simulink model "fec_ber_hw_V2"  (R2020b)
settings: Solver=FixedStepDiscrete  StartTime=0.0  StopTime=T  RelTol=1e-3
values from neighbouring files (symbols this model uses):
  aximm_awgn_reset = 0    [setup.m]
  aximm_bit_count_reset = 0    [setup.m]
  aximm_bits = n_blocks * k    (= 80)    [setup.m]
  aximm_ctrl_word_dec = 0    [setup.m]
  aximm_ctrl_word_enc = 0    [setup.m]
  aximm_enable = 1    [setup.m]
  aximm_length = k * n_blocks    (= 80)    [setup.m]
  aximm_length_dec = n    (= 160)    [setup.m]
  aximm_length_enc = k    (= 80)    [setup.m]
  aximm_llr_mag_reset = 0    [setup.m]
  aximm_llr_scale = (1/noise_var) * llr_scale    (= 1000)    [setup.m]
  aximm_load_dec = 1    [setup.m]
  aximm_load_enc = 1    [setup.m]
  aximm_noise_std = sqrt(noise_var)    [setup.m]
  aximm_reset = 0    [setup.m]
  d = sqrt(-2*log([0:1/4095:1]))    [setup.m]
  fs = 160e6    (= 160000000)    [setup.m]
  generator_polynomial = '''z^13 + z^12 + z^11 + z^8 + 1'''    [setup.m]
  llr_scale = 7.75/7.75    (= 1)    [setup.m]
libraries: simulink x931, hdlsllib x419, commseqgen3 x52, dspsigops x22, commblkcod2 x3, lib_rfsoc_fec x2
(part 4 of 47)

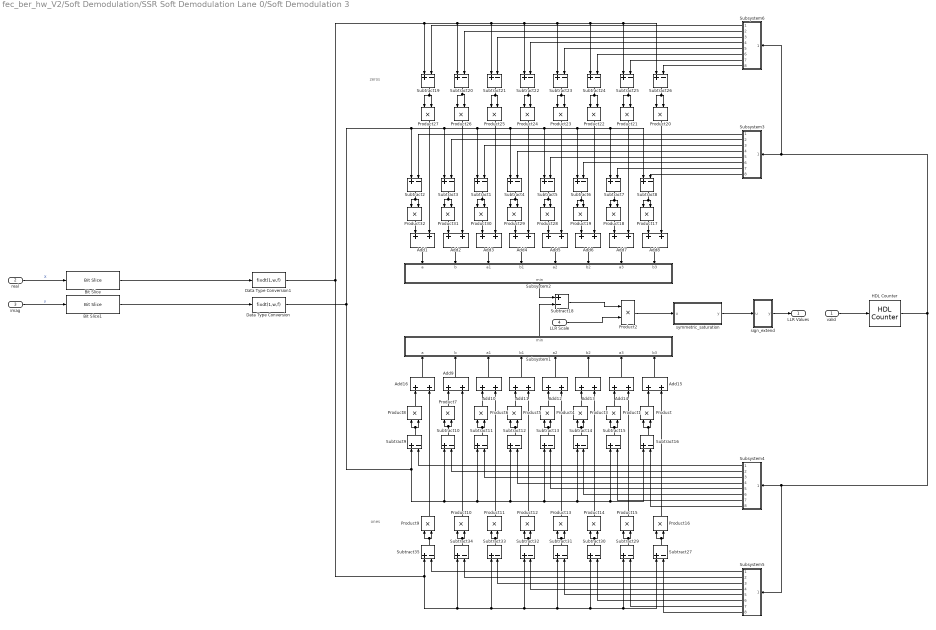
== system fec_ber_hw_V2/Soft Demodulation/SSR Soft Demodulation Lane 0/Soft Demodulation 3 ==
  note: ones
  note: zeros
  valid : Inport
  real : Inport  Port=2
  imag : Inport  Port=3
  LLR Scale : Inport  Port=4
  Add{1..16} (16 alike) : Sum  OutDataTypeStr=fixdt(1,(w+1)*2+1,f*2)  SaturateOnIntegerOverflow=on
  Bit Slice : hdlsllib/Logic and Bit Operations/Bit Slice  lidx=(n*w)-1  ridx=(n-1)*w
      settings: SourceProductBaseCode=SL
  Bit Slice1 : hdlsllib/Logic and Bit Operations/Bit Slice  lidx=(n*w)-1  ridx=(n-1)*w
      settings: SourceProductBaseCode=SL
  Data Type Conversion : DataTypeConversion  OutDataTypeStr=fixdt(1,w,f)  ConvertRealWorld=Stored Integer (SI)
  Data Type Conversion1 : DataTypeConversion  OutDataTypeStr=fixdt(1,w,f)  ConvertRealWorld=Stored Integer (SI)
  HDL Counter : hdlsllib/Sources/HDL Counter  CountType=Count limited  CountInit=0  CountStep=1  CountMax=3  CountFromType=Initial value  CountFrom=0  CountResetPort=off  CountLoadPort=off  CountEnbPort=on  CountDirPort=off  CountDataType=Unsigned  CountWordLen=2  CountFracLen=0  CountSampTime=1/(fs*2)
  Product{,1,3..16} (16 alike) : Product  SaturateOnIntegerOverflow=on
  Product{17..32} (16 alike) : Product
  Product2 : Product  RndMeth=Round  SaturateOnIntegerOverflow=on
  Subsystem1 : Subsystem
  Subsystem2 : Subsystem
  Subsystem3 : Subsystem
  Subsystem4 : Subsystem
  Subsystem5 : Subsystem
  Subsystem6 : Subsystem
  Subtract{1..16,19..27,29..35} (32 alike) : Sum  Inputs=+-  OutDataTypeStr=fixdt(1,w+1,f)  SaturateOnIntegerOverflow=on
  Subtract18 : Sum  Inputs=+-  OutDataTypeStr=fixdt(1,(w+1)*2+2,f*2)  SaturateOnIntegerOverflow=on
  sign_extend : Subsystem
  symmetric_saturation : MATLAB Function  TreatAsAtomicUnit=on
  LLR Values : Outport
  wires:
  Bit Slice/1 -> Data Type Conversion1/1
  Bit Slice1/1 -> Data Type Conversion/1
  Data Type Conversion1/1 -> Subtract27/1, Subtract29/1, Subtract30/1, Subtract31/1, Subtract32/1, Subtract33/1, Subtract34/1, Subtract35/1, Subtract20/1, Subtract26/1, Subtract25/1, Subtract24/1, Subtract23/1, Subtract22/1, Subtract21/1, Subtract19/1
  Data Type Conversion/1 -> Subtract15/1, Subtract16/1, Subtract14/1, Subtract13/1, Subtract12/1, Subtract11/1, Subtract10/1, Subtract9/1, Subtract7/1, Subtract8/1, Subtract6/1, Subtract5/1, Subtract4/1, Subtract1/1, Subtract3/1, Subtract2/1
  sign_extend/1(y) -> LLR Values/1
  Product2/1 -> symmetric_saturation/1(u)
  symmetric_saturation/1(y) -> sign_extend/1(u)
  HDL Counter/1 -> Subsystem3/1(enb), Subsystem6/1(enb), Subsystem4/1(enb), Subsystem5/1(enb)
  valid/1 -> HDL Counter/1
  Subsystem6/8(Out8) -> Subtract26/2
  Subsystem6/7(Out7) -> Subtract25/2
  Subsystem6/6(Out6) -> Subtract24/2
  Subsystem6/5(Out5) -> Subtract23/2
  Subsystem6/4(Out4) -> Subtract22/2
  Subsystem6/3(Out3) -> Subtract21/2
  Subsystem6/2(Out2) -> Subtract20/2
  Subsystem6/1(Out1) -> Subtract19/2
  Subtract6/1 -> Product19/2, Product19/1
  Subtract22/1 -> Product24/2, Product24/1
  Subtract20/1 -> Product26/1, Product26/2
  Subtract7/1 -> Product18/2, Product18/1
  Subtract8/1 -> Product17/1, Product17/2
  Subtract27/1 -> Product16/2, Product16/1
  Subtract29/1 -> Product15/2, Product15/1
  Subtract30/1 -> Product14/2, Product14/1
  Subtract31/1 -> Product13/2, Product13/1
  Subtract32/1 -> Product12/2, Product12/1
  Subtract33/1 -> Product11/2, Product11/1
  Subtract14/1 -> Product3/2, Product3/1
  Subsystem5/5(Out5) -> Subtract31/2
  Subtract16/1 -> Product/1, Product/2
  Add5/1 -> Subsystem2/5(a2)
  Subsystem3/8(Out8) -> Subtract8/2
  Add4/1 -> Subsystem2/4(b1)
  Product11/1 -> Add10/2
  Product29/1 -> Add4/1
  Subsystem4/8(Out8) -> Subtract16/2
  Subsystem4/2(Out2) -> Subtract10/2
  Subsystem5/8(Out8) -> Subtract27/2
  Subsystem5/7(Out7) -> Subtract29/2
  Subtract11/1 -> Product6/1, Product6/2
  Subtract34/1 -> Product10/1, Product10/2
  Product32/1 -> Add1/1
  Subsystem5/1(Out1) -> Subtract35/2
  Subtract12/1 -> Product5/1, Product5/2
  Subsystem3/7(Out7) -> Subtract7/2
  Product16/1 -> Add15/2
  Subsystem4/1(Out1) -> Subtract9/2
  Subsystem5/6(Out6) -> Subtract30/2
  Product24/1 -> Add4/2
  Subtract3/1 -> Product31/2, Product31/1
  Product13/1 -> Add12/2
  Subsystem5/3(Out3) -> Subtract33/2
  Subsystem5/2(Out2) -> Subtract34/2
  Subsystem4/3(Out3) -> Subtract11/2
  Product17/1 -> Add8/1
  Subsystem4/4(Out4) -> Subtract12/2
  Product9/1 -> Add16/2
  Add9/1 -> Subsystem1/2(b)
  Subsystem4/7(Out7) -> Subtract15/2
  Subtract26/1 -> Product20/2, Product20/1
  Subsystem3/3(Out3) -> Subtract1/2
  Product28/1 -> Add5/1
  Product12/1 -> Add11/2
  Product8/1 -> Add16/1
  Product7/1 -> Add9/1
  Subsystem4/5(Out5) -> Subtract13/2
  Subsystem3/4(Out4) -> Subtract4/2
  Product21/1 -> Add7/2
  Subtract25/1 -> Product21/2, Product21/1
  Add6/1 -> Subsystem2/6(b2)
  Add11/1 -> Subsystem1/4(b1)
  Add2/1 -> Subsystem2/2(b)
  Product15/1 -> Add14/2
  Product14/1 -> Add13/2
  Add8/1 -> Subsystem2/8(b3)
  Product27/1 -> Add1/2
  Subsystem3/1(Out1) -> Subtract2/2
  Subtract9/1 -> Product8/1, Product8/2
  Subtract15/1 -> Product1/1, Product1/2
  Subtract23/1 -> Product23/1, Product23/2
  Add14/1 -> Subsystem1/7(a3)
  imag/1 -> Bit Slice1/1  "y"
  Add16/1 -> Subsystem1/1(a)
  Subtract2/1 -> Product32/2, Product32/1
  Subtract5/1 -> Product28/2, Product28/1
  Subtract4/1 -> Product29/1, Product29/2
  Product18/1 -> Add7/1
  Add15/1 -> Subsystem1/8(b3)
  Product30/1 -> Add3/1
  Subsystem3/5(Out5) -> Subtract5/2
  Product31/1 -> Add2/1
  Subtract19/1 -> Product27/2, Product27/1
  Product26/1 -> Add2/2
  Add13/1 -> Subsystem1/6(b2)
  Subsystem3/2(Out2) -> Subtract3/2
  Product22/1 -> Add6/2
  Subsystem1/1(min) -> Subtract18/2
  Product5/1 -> Add11/1
  Subtract18/1 -> Product2/1
  Subsystem4/6(Out6) -> Subtract14/2
  Subtract1/1 -> Product30/2, Product30/1
  Subtract24/1 -> Product22/2, Product22/1
  Add10/1 -> Subsystem1/3(a1)
  LLR Scale/1 -> Product2/2
  Product4/1 -> Add12/1
  Subtract21/1 -> Product25/2, Product25/1
  Product23/1 -> Add5/2
  Add7/1 -> Subsystem2/7(a3)
  Product3/1 -> Add13/1
  Product19/1 -> Add6/1
  Product25/1 -> Add3/2
  real/1 -> Bit Slice/1  "X"
  Subtract35/1 -> Product9/1, Product9/2
  Subtract10/1 -> Product7/1, Product7/2
  Subsystem3/6(Out6) -> Subtract6/2
  Subsystem2/1(min) -> Subtract18/1
  Add3/1 -> Subsystem2/3(a1)
  Product20/1 -> Add8/2
  Add1/1 -> Subsystem2/1(a)
  Product/1 -> Add15/1
  Subtract13/1 -> Product4/2, Product4/1
  Product1/1 -> Add14/1
  Add12/1 -> Subsystem1/5(a2)
  Product10/1 -> Add9/2
  Product6/1 -> Add10/1
  Subsystem5/4(Out4) -> Subtract32/2

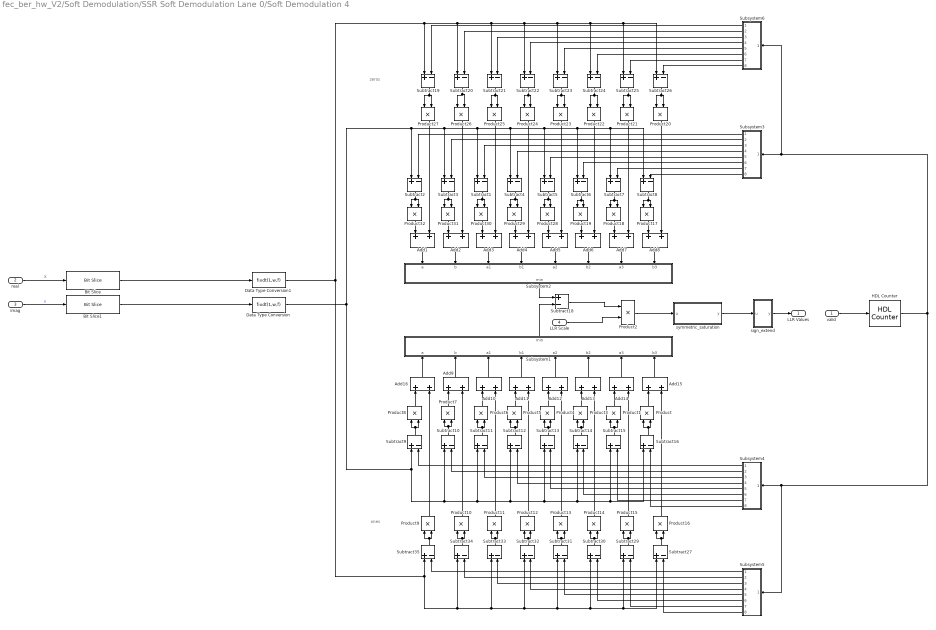
== system fec_ber_hw_V2/Soft Demodulation/SSR Soft Demodulation Lane 0/Soft Demodulation 4 ==
  note: ones
  note: zeros
  valid : Inport
  real : Inport  Port=2
  imag : Inport  Port=3
  LLR Scale : Inport  Port=4
  Add{1..16} (16 alike) : Sum  OutDataTypeStr=fixdt(1,(w+1)*2+1,f*2)  SaturateOnIntegerOverflow=on
  Bit Slice : hdlsllib/Logic and Bit Operations/Bit Slice  lidx=(n*w)-1  ridx=(n-1)*w
      settings: SourceProductBaseCode=SL
  Bit Slice1 : hdlsllib/Logic and Bit Operations/Bit Slice  lidx=(n*w)-1  ridx=(n-1)*w
      settings: SourceProductBaseCode=SL
  Data Type Conversion : DataTypeConversion  OutDataTypeStr=fixdt(1,w,f)  ConvertRealWorld=Stored Integer (SI)
  Data Type Conversion1 : DataTypeConversion  OutDataTypeStr=fixdt(1,w,f)  ConvertRealWorld=Stored Integer (SI)
  HDL Counter : hdlsllib/Sources/HDL Counter  CountType=Count limited  CountInit=0  CountStep=1  CountMax=3  CountFromType=Initial value  CountFrom=0  CountResetPort=off  CountLoadPort=off  CountEnbPort=on  CountDirPort=off  CountDataType=Unsigned  CountWordLen=2  CountFracLen=0  CountSampTime=1/(fs*2)
  Product{,1,3..16} (16 alike) : Product  SaturateOnIntegerOverflow=on
  Product{17..32} (16 alike) : Product
  Product2 : Product  RndMeth=Round  SaturateOnIntegerOverflow=on
  Subsystem1 : Subsystem
  Subsystem2 : Subsystem
  Subsystem3 : Subsystem
  Subsystem4 : Subsystem
  Subsystem5 : Subsystem
  Subsystem6 : Subsystem
  Subtract{1..16,19..27,29..35} (32 alike) : Sum  Inputs=+-  OutDataTypeStr=fixdt(1,w+1,f)  SaturateOnIntegerOverflow=on
  Subtract18 : Sum  Inputs=+-  OutDataTypeStr=fixdt(1,(w+1)*2+2,f*2)  SaturateOnIntegerOverflow=on
  sign_extend : Subsystem
  symmetric_saturation : MATLAB Function  TreatAsAtomicUnit=on
  LLR Values : Outport
  wires:
  Bit Slice/1 -> Data Type Conversion1/1
  Bit Slice1/1 -> Data Type Conversion/1
  Data Type Conversion1/1 -> Subtract27/1, Subtract29/1, Subtract30/1, Subtract31/1, Subtract32/1, Subtract33/1, Subtract34/1, Subtract35/1, Subtract20/1, Subtract26/1, Subtract25/1, Subtract24/1, Subtract23/1, Subtract22/1, Subtract21/1, Subtract19/1
  Data Type Conversion/1 -> Subtract15/1, Subtract16/1, Subtract14/1, Subtract13/1, Subtract12/1, Subtract11/1, Subtract10/1, Subtract9/1, Subtract7/1, Subtract8/1, Subtract6/1, Subtract5/1, Subtract4/1, Subtract1/1, Subtract3/1, Subtract2/1
  sign_extend/1(y) -> LLR Values/1
  Product2/1 -> symmetric_saturation/1(u)
  symmetric_saturation/1(y) -> sign_extend/1(u)
  HDL Counter/1 -> Subsystem3/1(enb), Subsystem6/1(enb), Subsystem4/1(enb), Subsystem5/1(enb)
  valid/1 -> HDL Counter/1
  Subsystem6/8(Out8) -> Subtract26/2
  Subsystem6/7(Out7) -> Subtract25/2
  Subsystem6/6(Out6) -> Subtract24/2
  Subsystem6/5(Out5) -> Subtract23/2
  Subsystem6/4(Out4) -> Subtract22/2
  Subsystem6/3(Out3) -> Subtract21/2
  Subsystem6/2(Out2) -> Subtract20/2
  Subsystem6/1(Out1) -> Subtract19/2
  Subtract6/1 -> Product19/2, Product19/1
  Subtract22/1 -> Product24/2, Product24/1
  Subtract20/1 -> Product26/1, Product26/2
  Subtract7/1 -> Product18/2, Product18/1
  Subtract8/1 -> Product17/1, Product17/2
  Subtract27/1 -> Product16/2, Product16/1
  Subtract29/1 -> Product15/2, Product15/1
  Subtract30/1 -> Product14/2, Product14/1
  Subtract31/1 -> Product13/2, Product13/1
  Subtract32/1 -> Product12/2, Product12/1
  Subtract33/1 -> Product11/2, Product11/1
  Subtract14/1 -> Product3/2, Product3/1
  Subsystem5/5(Out5) -> Subtract31/2
  Subtract16/1 -> Product/1, Product/2
  Add5/1 -> Subsystem2/5(a2)
  Subsystem3/8(Out8) -> Subtract8/2
  Add4/1 -> Subsystem2/4(b1)
  Product11/1 -> Add10/2
  Product29/1 -> Add4/1
  Subsystem4/8(Out8) -> Subtract16/2
  Subsystem4/2(Out2) -> Subtract10/2
  Subsystem5/8(Out8) -> Subtract27/2
  Subsystem5/7(Out7) -> Subtract29/2
  Subtract11/1 -> Product6/1, Product6/2
  Subtract34/1 -> Product10/1, Product10/2
  Product32/1 -> Add1/1
  Subsystem5/1(Out1) -> Subtract35/2
  Subtract12/1 -> Product5/1, Product5/2
  Subsystem3/7(Out7) -> Subtract7/2
  Product16/1 -> Add15/2
  Subsystem4/1(Out1) -> Subtract9/2
  Subsystem5/6(Out6) -> Subtract30/2
  Product24/1 -> Add4/2
  Subtract3/1 -> Product31/2, Product31/1
  Product13/1 -> Add12/2
  Subsystem5/3(Out3) -> Subtract33/2
  Subsystem5/2(Out2) -> Subtract34/2
  Subsystem4/3(Out3) -> Subtract11/2
  Product17/1 -> Add8/1
  Subsystem4/4(Out4) -> Subtract12/2
  Product9/1 -> Add16/2
  Add9/1 -> Subsystem1/2(b)
  Subsystem4/7(Out7) -> Subtract15/2
  Subtract26/1 -> Product20/2, Product20/1
  Subsystem3/3(Out3) -> Subtract1/2
  Product28/1 -> Add5/1
  Product12/1 -> Add11/2
  Product8/1 -> Add16/1
  Product7/1 -> Add9/1
  Subsystem4/5(Out5) -> Subtract13/2
  Subsystem3/4(Out4) -> Subtract4/2
  Product21/1 -> Add7/2
  Subtract25/1 -> Product21/2, Product21/1
  Add6/1 -> Subsystem2/6(b2)
  Add11/1 -> Subsystem1/4(b1)
  Add2/1 -> Subsystem2/2(b)
  Product15/1 -> Add14/2
  Product14/1 -> Add13/2
  Add8/1 -> Subsystem2/8(b3)
  Product27/1 -> Add1/2
  Subsystem3/1(Out1) -> Subtract2/2
  Subtract9/1 -> Product8/1, Product8/2
  Subtract15/1 -> Product1/1, Product1/2
  Subtract23/1 -> Product23/1, Product23/2
  Add14/1 -> Subsystem1/7(a3)
  imag/1 -> Bit Slice1/1  "y"
  Add16/1 -> Subsystem1/1(a)
  Subtract2/1 -> Product32/2, Product32/1
  Subtract5/1 -> Product28/2, Product28/1
  Subtract4/1 -> Product29/1, Product29/2
  Product18/1 -> Add7/1
  Add15/1 -> Subsystem1/8(b3)
  Product30/1 -> Add3/1
  Subsystem3/5(Out5) -> Subtract5/2
  Product31/1 -> Add2/1
  Subtract19/1 -> Product27/2, Product27/1
  Product26/1 -> Add2/2
  Add13/1 -> Subsystem1/6(b2)
  Subsystem3/2(Out2) -> Subtract3/2
  Product22/1 -> Add6/2
  Subsystem1/1(min) -> Subtract18/2
  Product5/1 -> Add11/1
  Subtract18/1 -> Product2/1
  Subsystem4/6(Out6) -> Subtract14/2
  Subtract1/1 -> Product30/2, Product30/1
  Subtract24/1 -> Product22/2, Product22/1
  Add10/1 -> Subsystem1/3(a1)
  LLR Scale/1 -> Product2/2
  Product4/1 -> Add12/1
  Subtract21/1 -> Product25/2, Product25/1
  Product23/1 -> Add5/2
  Add7/1 -> Subsystem2/7(a3)
  Product3/1 -> Add13/1
  Product19/1 -> Add6/1
  Product25/1 -> Add3/2
  real/1 -> Bit Slice/1  "X"
  Subtract35/1 -> Product9/1, Product9/2
  Subtract10/1 -> Product7/1, Product7/2
  Subsystem3/6(Out6) -> Subtract6/2
  Subsystem2/1(min) -> Subtract18/1
  Add3/1 -> Subsystem2/3(a1)
  Product20/1 -> Add8/2
  Add1/1 -> Subsystem2/1(a)
  Product/1 -> Add15/1
  Subtract13/1 -> Product4/2, Product4/1
  Product1/1 -> Add14/1
  Add12/1 -> Subsystem1/5(a2)
  Product10/1 -> Add9/2
  Product6/1 -> Add10/1
  Subsystem5/4(Out4) -> Subtract32/2

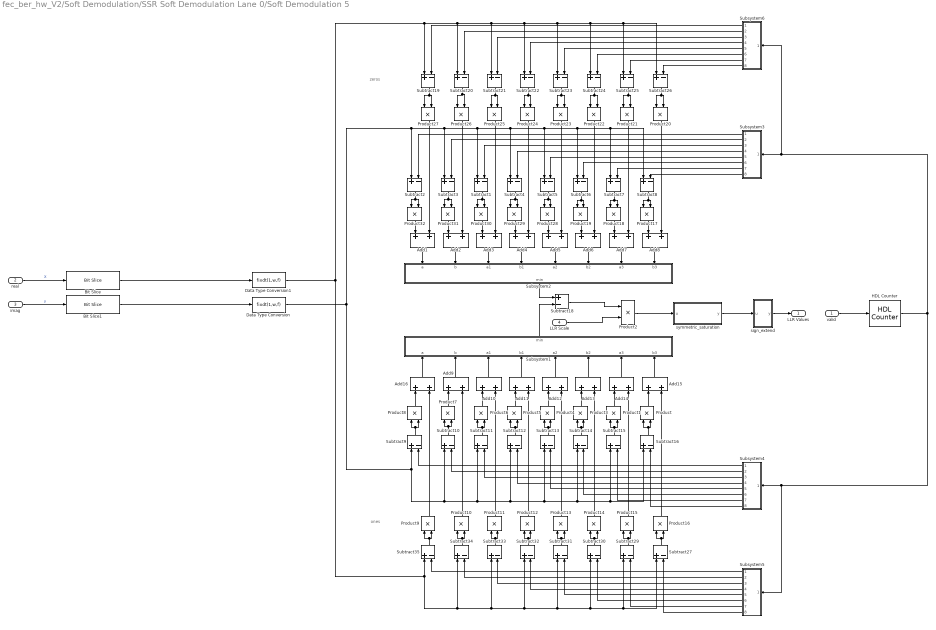
== system fec_ber_hw_V2/Soft Demodulation/SSR Soft Demodulation Lane 0/Soft Demodulation 5 ==
  note: ones
  note: zeros
  valid : Inport
  real : Inport  Port=2
  imag : Inport  Port=3
  LLR Scale : Inport  Port=4
  Add{1..16} (16 alike) : Sum  OutDataTypeStr=fixdt(1,(w+1)*2+1,f*2)  SaturateOnIntegerOverflow=on
  Bit Slice : hdlsllib/Logic and Bit Operations/Bit Slice  lidx=(n*w)-1  ridx=(n-1)*w
      settings: SourceProductBaseCode=SL
  Bit Slice1 : hdlsllib/Logic and Bit Operations/Bit Slice  lidx=(n*w)-1  ridx=(n-1)*w
      settings: SourceProductBaseCode=SL
  Data Type Conversion : DataTypeConversion  OutDataTypeStr=fixdt(1,w,f)  ConvertRealWorld=Stored Integer (SI)
  Data Type Conversion1 : DataTypeConversion  OutDataTypeStr=fixdt(1,w,f)  ConvertRealWorld=Stored Integer (SI)
  HDL Counter : hdlsllib/Sources/HDL Counter  CountType=Count limited  CountInit=0  CountStep=1  CountMax=3  CountFromType=Initial value  CountFrom=0  CountResetPort=off  CountLoadPort=off  CountEnbPort=on  CountDirPort=off  CountDataType=Unsigned  CountWordLen=2  CountFracLen=0  CountSampTime=1/(fs*2)
  Product{,1,3..16} (16 alike) : Product  SaturateOnIntegerOverflow=on
  Product{17..32} (16 alike) : Product
  Product2 : Product  RndMeth=Round  SaturateOnIntegerOverflow=on
  Subsystem1 : Subsystem
  Subsystem2 : Subsystem
  Subsystem3 : Subsystem
  Subsystem4 : Subsystem
  Subsystem5 : Subsystem
  Subsystem6 : Subsystem
  Subtract{1..16,19..27,29..35} (32 alike) : Sum  Inputs=+-  OutDataTypeStr=fixdt(1,w+1,f)  SaturateOnIntegerOverflow=on
  Subtract18 : Sum  Inputs=+-  OutDataTypeStr=fixdt(1,(w+1)*2+2,f*2)  SaturateOnIntegerOverflow=on
  sign_extend : Subsystem
  symmetric_saturation : MATLAB Function  TreatAsAtomicUnit=on
  LLR Values : Outport
  wires:
  Bit Slice/1 -> Data Type Conversion1/1
  Bit Slice1/1 -> Data Type Conversion/1
  Data Type Conversion1/1 -> Subtract27/1, Subtract29/1, Subtract30/1, Subtract31/1, Subtract32/1, Subtract33/1, Subtract34/1, Subtract35/1, Subtract20/1, Subtract26/1, Subtract25/1, Subtract24/1, Subtract23/1, Subtract22/1, Subtract21/1, Subtract19/1
  Data Type Conversion/1 -> Subtract15/1, Subtract16/1, Subtract14/1, Subtract13/1, Subtract12/1, Subtract11/1, Subtract10/1, Subtract9/1, Subtract7/1, Subtract8/1, Subtract6/1, Subtract5/1, Subtract4/1, Subtract1/1, Subtract3/1, Subtract2/1
  sign_extend/1(y) -> LLR Values/1
  Product2/1 -> symmetric_saturation/1(u)
  symmetric_saturation/1(y) -> sign_extend/1(u)
  HDL Counter/1 -> Subsystem3/1(enb), Subsystem6/1(enb), Subsystem4/1(enb), Subsystem5/1(enb)
  valid/1 -> HDL Counter/1
  Subsystem6/8(Out8) -> Subtract26/2
  Subsystem6/7(Out7) -> Subtract25/2
  Subsystem6/6(Out6) -> Subtract24/2
  Subsystem6/5(Out5) -> Subtract23/2
  Subsystem6/4(Out4) -> Subtract22/2
  Subsystem6/3(Out3) -> Subtract21/2
  Subsystem6/2(Out2) -> Subtract20/2
  Subsystem6/1(Out1) -> Subtract19/2
  Subtract6/1 -> Product19/2, Product19/1
  Subtract22/1 -> Product24/2, Product24/1
  Subtract20/1 -> Product26/1, Product26/2
  Subtract7/1 -> Product18/2, Product18/1
  Subtract8/1 -> Product17/1, Product17/2
  Subtract27/1 -> Product16/2, Product16/1
  Subtract29/1 -> Product15/2, Product15/1
  Subtract30/1 -> Product14/2, Product14/1
  Subtract31/1 -> Product13/2, Product13/1
  Subtract32/1 -> Product12/2, Product12/1
  Subtract33/1 -> Product11/2, Product11/1
  Subtract14/1 -> Product3/2, Product3/1
  Subsystem5/5(Out5) -> Subtract31/2
  Subtract16/1 -> Product/1, Product/2
  Add5/1 -> Subsystem2/5(a2)
  Subsystem3/8(Out8) -> Subtract8/2
  Add4/1 -> Subsystem2/4(b1)
  Product11/1 -> Add10/2
  Product29/1 -> Add4/1
  Subsystem4/8(Out8) -> Subtract16/2
  Subsystem4/2(Out2) -> Subtract10/2
  Subsystem5/8(Out8) -> Subtract27/2
  Subsystem5/7(Out7) -> Subtract29/2
  Subtract11/1 -> Product6/1, Product6/2
  Subtract34/1 -> Product10/1, Product10/2
  Product32/1 -> Add1/1
  Subsystem5/1(Out1) -> Subtract35/2
  Subtract12/1 -> Product5/1, Product5/2
  Subsystem3/7(Out7) -> Subtract7/2
  Product16/1 -> Add15/2
  Subsystem4/1(Out1) -> Subtract9/2
  Subsystem5/6(Out6) -> Subtract30/2
  Product24/1 -> Add4/2
  Subtract3/1 -> Product31/2, Product31/1
  Product13/1 -> Add12/2
  Subsystem5/3(Out3) -> Subtract33/2
  Subsystem5/2(Out2) -> Subtract34/2
  Subsystem4/3(Out3) -> Subtract11/2
  Product17/1 -> Add8/1
  Subsystem4/4(Out4) -> Subtract12/2
  Product9/1 -> Add16/2
  Add9/1 -> Subsystem1/2(b)
  Subsystem4/7(Out7) -> Subtract15/2
  Subtract26/1 -> Product20/2, Product20/1
  Subsystem3/3(Out3) -> Subtract1/2
  Product28/1 -> Add5/1
  Product12/1 -> Add11/2
  Product8/1 -> Add16/1
  Product7/1 -> Add9/1
  Subsystem4/5(Out5) -> Subtract13/2
  Subsystem3/4(Out4) -> Subtract4/2
  Product21/1 -> Add7/2
  Subtract25/1 -> Product21/2, Product21/1
  Add6/1 -> Subsystem2/6(b2)
  Add11/1 -> Subsystem1/4(b1)
  Add2/1 -> Subsystem2/2(b)
  Product15/1 -> Add14/2
  Product14/1 -> Add13/2
  Add8/1 -> Subsystem2/8(b3)
  Product27/1 -> Add1/2
  Subsystem3/1(Out1) -> Subtract2/2
  Subtract9/1 -> Product8/1, Product8/2
  Subtract15/1 -> Product1/1, Product1/2
  Subtract23/1 -> Product23/1, Product23/2
  Add14/1 -> Subsystem1/7(a3)
  imag/1 -> Bit Slice1/1  "y"
  Add16/1 -> Subsystem1/1(a)
  Subtract2/1 -> Product32/2, Product32/1
  Subtract5/1 -> Product28/2, Product28/1
  Subtract4/1 -> Product29/1, Product29/2
  Product18/1 -> Add7/1
  Add15/1 -> Subsystem1/8(b3)
  Product30/1 -> Add3/1
  Subsystem3/5(Out5) -> Subtract5/2
  Product31/1 -> Add2/1
  Subtract19/1 -> Product27/2, Product27/1
  Product26/1 -> Add2/2
  Add13/1 -> Subsystem1/6(b2)
  Subsystem3/2(Out2) -> Subtract3/2
  Product22/1 -> Add6/2
  Subsystem1/1(min) -> Subtract18/2
  Product5/1 -> Add11/1
  Subtract18/1 -> Product2/1
  Subsystem4/6(Out6) -> Subtract14/2
  Subtract1/1 -> Product30/2, Product30/1
  Subtract24/1 -> Product22/2, Product22/1
  Add10/1 -> Subsystem1/3(a1)
  LLR Scale/1 -> Product2/2
  Product4/1 -> Add12/1
  Subtract21/1 -> Product25/2, Product25/1
  Product23/1 -> Add5/2
  Add7/1 -> Subsystem2/7(a3)
  Product3/1 -> Add13/1
  Product19/1 -> Add6/1
  Product25/1 -> Add3/2
  real/1 -> Bit Slice/1  "X"
  Subtract35/1 -> Product9/1, Product9/2
  Subtract10/1 -> Product7/1, Product7/2
  Subsystem3/6(Out6) -> Subtract6/2
  Subsystem2/1(min) -> Subtract18/1
  Add3/1 -> Subsystem2/3(a1)
  Product20/1 -> Add8/2
  Add1/1 -> Subsystem2/1(a)
  Product/1 -> Add15/1
  Subtract13/1 -> Product4/2, Product4/1
  Product1/1 -> Add14/1
  Add12/1 -> Subsystem1/5(a2)
  Product10/1 -> Add9/2
  Product6/1 -> Add10/1
  Subsystem5/4(Out4) -> Subtract32/2

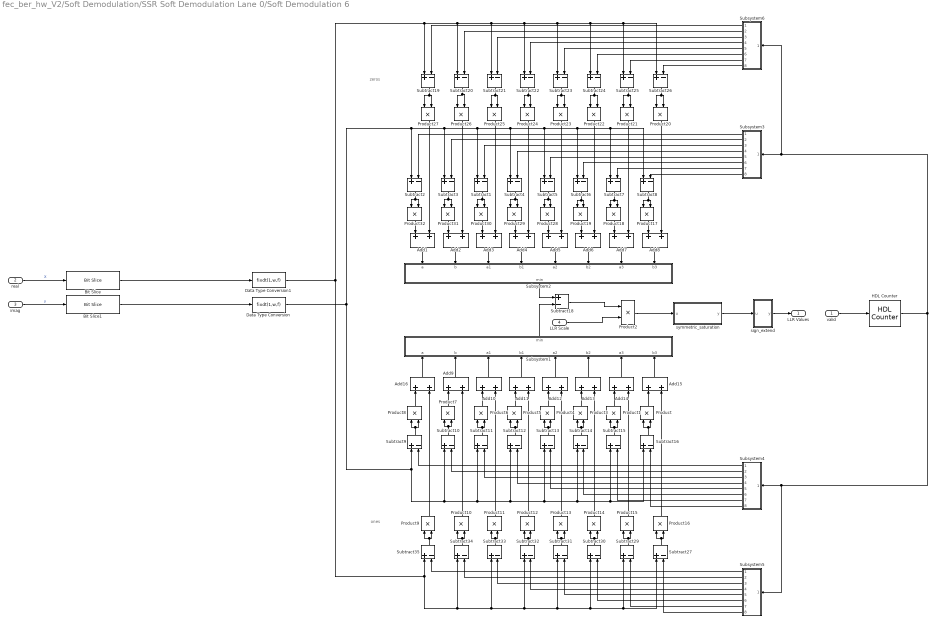
== system fec_ber_hw_V2/Soft Demodulation/SSR Soft Demodulation Lane 0/Soft Demodulation 6 ==
  note: ones
  note: zeros
  valid : Inport
  real : Inport  Port=2
  imag : Inport  Port=3
  LLR Scale : Inport  Port=4
  Add{1..16} (16 alike) : Sum  OutDataTypeStr=fixdt(1,(w+1)*2+1,f*2)  SaturateOnIntegerOverflow=on
  Bit Slice : hdlsllib/Logic and Bit Operations/Bit Slice  lidx=(n*w)-1  ridx=(n-1)*w
      settings: SourceProductBaseCode=SL
  Bit Slice1 : hdlsllib/Logic and Bit Operations/Bit Slice  lidx=(n*w)-1  ridx=(n-1)*w
      settings: SourceProductBaseCode=SL
  Data Type Conversion : DataTypeConversion  OutDataTypeStr=fixdt(1,w,f)  ConvertRealWorld=Stored Integer (SI)
  Data Type Conversion1 : DataTypeConversion  OutDataTypeStr=fixdt(1,w,f)  ConvertRealWorld=Stored Integer (SI)
  HDL Counter : hdlsllib/Sources/HDL Counter  CountType=Count limited  CountInit=0  CountStep=1  CountMax=3  CountFromType=Initial value  CountFrom=0  CountResetPort=off  CountLoadPort=off  CountEnbPort=on  CountDirPort=off  CountDataType=Unsigned  CountWordLen=2  CountFracLen=0  CountSampTime=1/(fs*2)
  Product{,1,3..16} (16 alike) : Product  SaturateOnIntegerOverflow=on
  Product{17..32} (16 alike) : Product
  Product2 : Product  RndMeth=Round  SaturateOnIntegerOverflow=on
  Subsystem1 : Subsystem
  Subsystem2 : Subsystem
  Subsystem3 : Subsystem
  Subsystem4 : Subsystem
  Subsystem5 : Subsystem
  Subsystem6 : Subsystem
  Subtract{1..16,19..27,29..35} (32 alike) : Sum  Inputs=+-  OutDataTypeStr=fixdt(1,w+1,f)  SaturateOnIntegerOverflow=on
  Subtract18 : Sum  Inputs=+-  OutDataTypeStr=fixdt(1,(w+1)*2+2,f*2)  SaturateOnIntegerOverflow=on
  sign_extend : Subsystem
  symmetric_saturation : MATLAB Function  TreatAsAtomicUnit=on
  LLR Values : Outport
  wires:
  Bit Slice/1 -> Data Type Conversion1/1
  Bit Slice1/1 -> Data Type Conversion/1
  Data Type Conversion1/1 -> Subtract27/1, Subtract29/1, Subtract30/1, Subtract31/1, Subtract32/1, Subtract33/1, Subtract34/1, Subtract35/1, Subtract20/1, Subtract26/1, Subtract25/1, Subtract24/1, Subtract23/1, Subtract22/1, Subtract21/1, Subtract19/1
  Data Type Conversion/1 -> Subtract15/1, Subtract16/1, Subtract14/1, Subtract13/1, Subtract12/1, Subtract11/1, Subtract10/1, Subtract9/1, Subtract7/1, Subtract8/1, Subtract6/1, Subtract5/1, Subtract4/1, Subtract1/1, Subtract3/1, Subtract2/1
  sign_extend/1(y) -> LLR Values/1
  Product2/1 -> symmetric_saturation/1(u)
  symmetric_saturation/1(y) -> sign_extend/1(u)
  HDL Counter/1 -> Subsystem3/1(enb), Subsystem6/1(enb), Subsystem4/1(enb), Subsystem5/1(enb)
  valid/1 -> HDL Counter/1
  Subsystem6/8(Out8) -> Subtract26/2
  Subsystem6/7(Out7) -> Subtract25/2
  Subsystem6/6(Out6) -> Subtract24/2
  Subsystem6/5(Out5) -> Subtract23/2
  Subsystem6/4(Out4) -> Subtract22/2
  Subsystem6/3(Out3) -> Subtract21/2
  Subsystem6/2(Out2) -> Subtract20/2
  Subsystem6/1(Out1) -> Subtract19/2
  Subtract6/1 -> Product19/2, Product19/1
  Subtract22/1 -> Product24/2, Product24/1
  Subtract20/1 -> Product26/1, Product26/2
  Subtract7/1 -> Product18/2, Product18/1
  Subtract8/1 -> Product17/1, Product17/2
  Subtract27/1 -> Product16/2, Product16/1
  Subtract29/1 -> Product15/2, Product15/1
  Subtract30/1 -> Product14/2, Product14/1
  Subtract31/1 -> Product13/2, Product13/1
  Subtract32/1 -> Product12/2, Product12/1
  Subtract33/1 -> Product11/2, Product11/1
  Subtract14/1 -> Product3/2, Product3/1
  Subsystem5/5(Out5) -> Subtract31/2
  Subtract16/1 -> Product/1, Product/2
  Add5/1 -> Subsystem2/5(a2)
  Subsystem3/8(Out8) -> Subtract8/2
  Add4/1 -> Subsystem2/4(b1)
  Product11/1 -> Add10/2
  Product29/1 -> Add4/1
  Subsystem4/8(Out8) -> Subtract16/2
  Subsystem4/2(Out2) -> Subtract10/2
  Subsystem5/8(Out8) -> Subtract27/2
  Subsystem5/7(Out7) -> Subtract29/2
  Subtract11/1 -> Product6/1, Product6/2
  Subtract34/1 -> Product10/1, Product10/2
  Product32/1 -> Add1/1
  Subsystem5/1(Out1) -> Subtract35/2
  Subtract12/1 -> Product5/1, Product5/2
  Subsystem3/7(Out7) -> Subtract7/2
  Product16/1 -> Add15/2
  Subsystem4/1(Out1) -> Subtract9/2
  Subsystem5/6(Out6) -> Subtract30/2
  Product24/1 -> Add4/2
  Subtract3/1 -> Product31/2, Product31/1
  Product13/1 -> Add12/2
  Subsystem5/3(Out3) -> Subtract33/2
  Subsystem5/2(Out2) -> Subtract34/2
  Subsystem4/3(Out3) -> Subtract11/2
  Product17/1 -> Add8/1
  Subsystem4/4(Out4) -> Subtract12/2
  Product9/1 -> Add16/2
  Add9/1 -> Subsystem1/2(b)
  Subsystem4/7(Out7) -> Subtract15/2
  Subtract26/1 -> Product20/2, Product20/1
  Subsystem3/3(Out3) -> Subtract1/2
  Product28/1 -> Add5/1
  Product12/1 -> Add11/2
  Product8/1 -> Add16/1
  Product7/1 -> Add9/1
  Subsystem4/5(Out5) -> Subtract13/2
  Subsystem3/4(Out4) -> Subtract4/2
  Product21/1 -> Add7/2
  Subtract25/1 -> Product21/2, Product21/1
  Add6/1 -> Subsystem2/6(b2)
  Add11/1 -> Subsystem1/4(b1)
  Add2/1 -> Subsystem2/2(b)
  Product15/1 -> Add14/2
  Product14/1 -> Add13/2
  Add8/1 -> Subsystem2/8(b3)
  Product27/1 -> Add1/2
  Subsystem3/1(Out1) -> Subtract2/2
  Subtract9/1 -> Product8/1, Product8/2
  Subtract15/1 -> Product1/1, Product1/2
  Subtract23/1 -> Product23/1, Product23/2
  Add14/1 -> Subsystem1/7(a3)
  imag/1 -> Bit Slice1/1  "y"
  Add16/1 -> Subsystem1/1(a)
  Subtract2/1 -> Product32/2, Product32/1
  Subtract5/1 -> Product28/2, Product28/1
  Subtract4/1 -> Product29/1, Product29/2
  Product18/1 -> Add7/1
  Add15/1 -> Subsystem1/8(b3)
  Product30/1 -> Add3/1
  Subsystem3/5(Out5) -> Subtract5/2
  Product31/1 -> Add2/1
  Subtract19/1 -> Product27/2, Product27/1
  Product26/1 -> Add2/2
  Add13/1 -> Subsystem1/6(b2)
  Subsystem3/2(Out2) -> Subtract3/2
  Product22/1 -> Add6/2
  Subsystem1/1(min) -> Subtract18/2
  Product5/1 -> Add11/1
  Subtract18/1 -> Product2/1
  Subsystem4/6(Out6) -> Subtract14/2
  Subtract1/1 -> Product30/2, Product30/1
  Subtract24/1 -> Product22/2, Product22/1
  Add10/1 -> Subsystem1/3(a1)
  LLR Scale/1 -> Product2/2
  Product4/1 -> Add12/1
  Subtract21/1 -> Product25/2, Product25/1
  Product23/1 -> Add5/2
  Add7/1 -> Subsystem2/7(a3)
  Product3/1 -> Add13/1
  Product19/1 -> Add6/1
  Product25/1 -> Add3/2
  real/1 -> Bit Slice/1  "X"
  Subtract35/1 -> Product9/1, Product9/2
  Subtract10/1 -> Product7/1, Product7/2
  Subsystem3/6(Out6) -> Subtract6/2
  Subsystem2/1(min) -> Subtract18/1
  Add3/1 -> Subsystem2/3(a1)
  Product20/1 -> Add8/2
  Add1/1 -> Subsystem2/1(a)
  Product/1 -> Add15/1
  Subtract13/1 -> Product4/2, Product4/1
  Product1/1 -> Add14/1
  Add12/1 -> Subsystem1/5(a2)
  Product10/1 -> Add9/2
  Product6/1 -> Add10/1
  Subsystem5/4(Out4) -> Subtract32/2

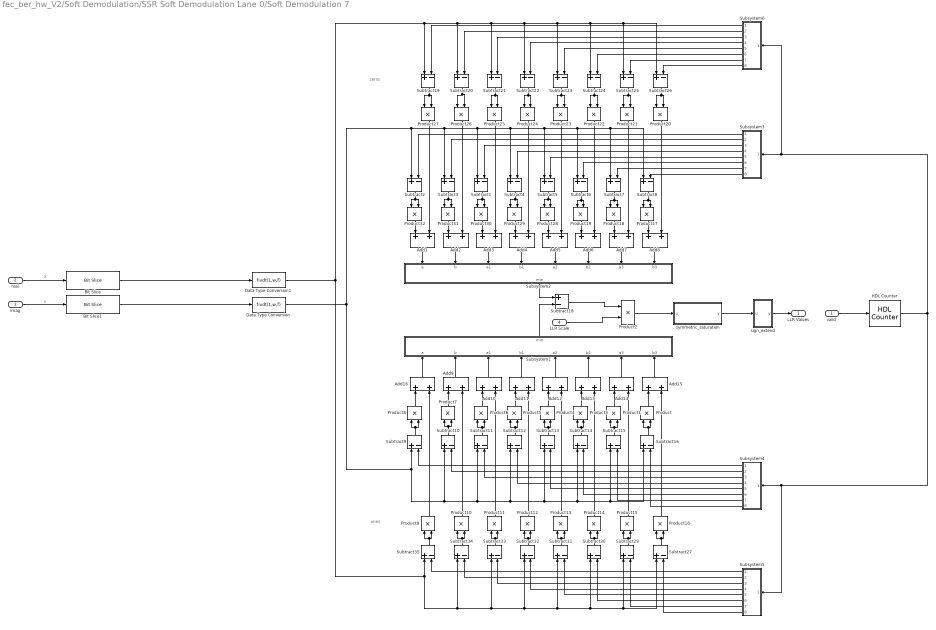
== system fec_ber_hw_V2/Soft Demodulation/SSR Soft Demodulation Lane 0/Soft Demodulation 7 ==
  note: ones
  note: zeros
  valid : Inport
  real : Inport  Port=2
  imag : Inport  Port=3
  LLR Scale : Inport  Port=4
  Add{1..16} (16 alike) : Sum  OutDataTypeStr=fixdt(1,(w+1)*2+1,f*2)  SaturateOnIntegerOverflow=on
  Bit Slice : hdlsllib/Logic and Bit Operations/Bit Slice  lidx=(n*w)-1  ridx=(n-1)*w
      settings: SourceProductBaseCode=SL
  Bit Slice1 : hdlsllib/Logic and Bit Operations/Bit Slice  lidx=(n*w)-1  ridx=(n-1)*w
      settings: SourceProductBaseCode=SL
  Data Type Conversion : DataTypeConversion  OutDataTypeStr=fixdt(1,w,f)  ConvertRealWorld=Stored Integer (SI)
  Data Type Conversion1 : DataTypeConversion  OutDataTypeStr=fixdt(1,w,f)  ConvertRealWorld=Stored Integer (SI)
  HDL Counter : hdlsllib/Sources/HDL Counter  CountType=Count limited  CountInit=0  CountStep=1  CountMax=3  CountFromType=Initial value  CountFrom=0  CountResetPort=off  CountLoadPort=off  CountEnbPort=on  CountDirPort=off  CountDataType=Unsigned  CountWordLen=2  CountFracLen=0  CountSampTime=1/(fs*2)
  Product{,1,3..16} (16 alike) : Product  SaturateOnIntegerOverflow=on
  Product{17..32} (16 alike) : Product
  Product2 : Product  RndMeth=Round  SaturateOnIntegerOverflow=on
  Subsystem1 : Subsystem
  Subsystem2 : Subsystem
  Subsystem3 : Subsystem
  Subsystem4 : Subsystem
  Subsystem5 : Subsystem
  Subsystem6 : Subsystem
  Subtract{1..16,19..27,29..35} (32 alike) : Sum  Inputs=+-  OutDataTypeStr=fixdt(1,w+1,f)  SaturateOnIntegerOverflow=on
  Subtract18 : Sum  Inputs=+-  OutDataTypeStr=fixdt(1,(w+1)*2+2,f*2)  SaturateOnIntegerOverflow=on
  sign_extend : Subsystem
  symmetric_saturation : MATLAB Function  TreatAsAtomicUnit=on
  LLR Values : Outport
  wires:
  Bit Slice/1 -> Data Type Conversion1/1
  Bit Slice1/1 -> Data Type Conversion/1
  Data Type Conversion1/1 -> Subtract27/1, Subtract29/1, Subtract30/1, Subtract31/1, Subtract32/1, Subtract33/1, Subtract34/1, Subtract35/1, Subtract20/1, Subtract26/1, Subtract25/1, Subtract24/1, Subtract23/1, Subtract22/1, Subtract21/1, Subtract19/1
  Data Type Conversion/1 -> Subtract15/1, Subtract16/1, Subtract14/1, Subtract13/1, Subtract12/1, Subtract11/1, Subtract10/1, Subtract9/1, Subtract7/1, Subtract8/1, Subtract6/1, Subtract5/1, Subtract4/1, Subtract1/1, Subtract3/1, Subtract2/1
  sign_extend/1(y) -> LLR Values/1
  Product2/1 -> symmetric_saturation/1(u)
  symmetric_saturation/1(y) -> sign_extend/1(u)
  HDL Counter/1 -> Subsystem3/1(enb), Subsystem6/1(enb), Subsystem4/1(enb), Subsystem5/1(enb)
  valid/1 -> HDL Counter/1
  Subsystem6/8(Out8) -> Subtract26/2
  Subsystem6/7(Out7) -> Subtract25/2
  Subsystem6/6(Out6) -> Subtract24/2
  Subsystem6/5(Out5) -> Subtract23/2
  Subsystem6/4(Out4) -> Subtract22/2
  Subsystem6/3(Out3) -> Subtract21/2
  Subsystem6/2(Out2) -> Subtract20/2
  Subsystem6/1(Out1) -> Subtract19/2
  Subtract6/1 -> Product19/2, Product19/1
  Subtract22/1 -> Product24/2, Product24/1
  Subtract20/1 -> Product26/1, Product26/2
  Subtract7/1 -> Product18/2, Product18/1
  Subtract8/1 -> Product17/1, Product17/2
  Subtract27/1 -> Product16/2, Product16/1
  Subtract29/1 -> Product15/2, Product15/1
  Subtract30/1 -> Product14/2, Product14/1
  Subtract31/1 -> Product13/2, Product13/1
  Subtract32/1 -> Product12/2, Product12/1
  Subtract33/1 -> Product11/2, Product11/1
  Subtract14/1 -> Product3/2, Product3/1
  Subsystem5/5(Out5) -> Subtract31/2
  Subtract16/1 -> Product/1, Product/2
  Add5/1 -> Subsystem2/5(a2)
  Subsystem3/8(Out8) -> Subtract8/2
  Add4/1 -> Subsystem2/4(b1)
  Product11/1 -> Add10/2
  Product29/1 -> Add4/1
  Subsystem4/8(Out8) -> Subtract16/2
  Subsystem4/2(Out2) -> Subtract10/2
  Subsystem5/8(Out8) -> Subtract27/2
  Subsystem5/7(Out7) -> Subtract29/2
  Subtract11/1 -> Product6/1, Product6/2
  Subtract34/1 -> Product10/1, Product10/2
  Product32/1 -> Add1/1
  Subsystem5/1(Out1) -> Subtract35/2
  Subtract12/1 -> Product5/1, Product5/2
  Subsystem3/7(Out7) -> Subtract7/2
  Product16/1 -> Add15/2
  Subsystem4/1(Out1) -> Subtract9/2
  Subsystem5/6(Out6) -> Subtract30/2
  Product24/1 -> Add4/2
  Subtract3/1 -> Product31/2, Product31/1
  Product13/1 -> Add12/2
  Subsystem5/3(Out3) -> Subtract33/2
  Subsystem5/2(Out2) -> Subtract34/2
  Subsystem4/3(Out3) -> Subtract11/2
  Product17/1 -> Add8/1
  Subsystem4/4(Out4) -> Subtract12/2
  Product9/1 -> Add16/2
  Add9/1 -> Subsystem1/2(b)
  Subsystem4/7(Out7) -> Subtract15/2
  Subtract26/1 -> Product20/2, Product20/1
  Subsystem3/3(Out3) -> Subtract1/2
  Product28/1 -> Add5/1
  Product12/1 -> Add11/2
  Product8/1 -> Add16/1
  Product7/1 -> Add9/1
  Subsystem4/5(Out5) -> Subtract13/2
  Subsystem3/4(Out4) -> Subtract4/2
  Product21/1 -> Add7/2
  Subtract25/1 -> Product21/2, Product21/1
  Add6/1 -> Subsystem2/6(b2)
  Add11/1 -> Subsystem1/4(b1)
  Add2/1 -> Subsystem2/2(b)
  Product15/1 -> Add14/2
  Product14/1 -> Add13/2
  Add8/1 -> Subsystem2/8(b3)
  Product27/1 -> Add1/2
  Subsystem3/1(Out1) -> Subtract2/2
  Subtract9/1 -> Product8/1, Product8/2
  Subtract15/1 -> Product1/1, Product1/2
  Subtract23/1 -> Product23/1, Product23/2
  Add14/1 -> Subsystem1/7(a3)
  imag/1 -> Bit Slice1/1  "y"
  Add16/1 -> Subsystem1/1(a)
  Subtract2/1 -> Product32/2, Product32/1
  Subtract5/1 -> Product28/2, Product28/1
  Subtract4/1 -> Product29/1, Product29/2
  Product18/1 -> Add7/1
  Add15/1 -> Subsystem1/8(b3)
  Product30/1 -> Add3/1
  Subsystem3/5(Out5) -> Subtract5/2
  Product31/1 -> Add2/1
  Subtract19/1 -> Product27/2, Product27/1
  Product26/1 -> Add2/2
  Add13/1 -> Subsystem1/6(b2)
  Subsystem3/2(Out2) -> Subtract3/2
  Product22/1 -> Add6/2
  Subsystem1/1(min) -> Subtract18/2
  Product5/1 -> Add11/1
  Subtract18/1 -> Product2/1
  Subsystem4/6(Out6) -> Subtract14/2
  Subtract1/1 -> Product30/2, Product30/1
  Subtract24/1 -> Product22/2, Product22/1
  Add10/1 -> Subsystem1/3(a1)
  LLR Scale/1 -> Product2/2
  Product4/1 -> Add12/1
  Subtract21/1 -> Product25/2, Product25/1
  Product23/1 -> Add5/2
  Add7/1 -> Subsystem2/7(a3)
  Product3/1 -> Add13/1
  Product19/1 -> Add6/1
  Product25/1 -> Add3/2
  real/1 -> Bit Slice/1  "X"
  Subtract35/1 -> Product9/1, Product9/2
  Subtract10/1 -> Product7/1, Product7/2
  Subsystem3/6(Out6) -> Subtract6/2
  Subsystem2/1(min) -> Subtract18/1
  Add3/1 -> Subsystem2/3(a1)
  Product20/1 -> Add8/2
  Add1/1 -> Subsystem2/1(a)
  Product/1 -> Add15/1
  Subtract13/1 -> Product4/2, Product4/1
  Product1/1 -> Add14/1
  Add12/1 -> Subsystem1/5(a2)
  Product10/1 -> Add9/2
  Product6/1 -> Add10/1
  Subsystem5/4(Out4) -> Subtract32/2

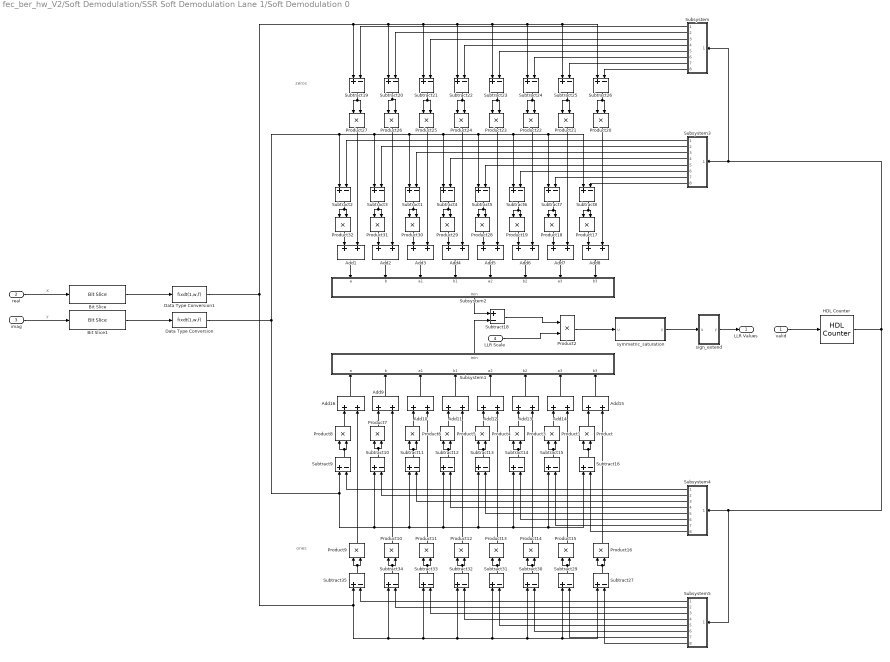
== system fec_ber_hw_V2/Soft Demodulation/SSR Soft Demodulation Lane 1/Soft Demodulation 0 ==
  note: ones
  note: zeros
  valid : Inport
  real : Inport  Port=2
  imag : Inport  Port=3
  LLR Scale : Inport  Port=4
  Add{1..16} (16 alike) : Sum  OutDataTypeStr=fixdt(1,(w+1)*2+1,f*2)  SaturateOnIntegerOverflow=on
  Bit Slice : hdlsllib/Logic and Bit Operations/Bit Slice  lidx=(n*w)-1  ridx=(n-1)*w
      settings: SourceProductBaseCode=SL
  Bit Slice1 : hdlsllib/Logic and Bit Operations/Bit Slice  lidx=(n*w)-1  ridx=(n-1)*w
      settings: SourceProductBaseCode=SL
  Data Type Conversion : DataTypeConversion  OutDataTypeStr=fixdt(1,w,f)  ConvertRealWorld=Stored Integer (SI)  SaturateOnIntegerOverflow=on
  Data Type Conversion1 : DataTypeConversion  OutDataTypeStr=fixdt(1,w,f)  ConvertRealWorld=Stored Integer (SI)  SaturateOnIntegerOverflow=on
  HDL Counter : hdlsllib/Sources/HDL Counter  CountType=Count limited  CountInit=0  CountStep=1  CountMax=3  CountFromType=Initial value  CountFrom=0  CountResetPort=off  CountLoadPort=off  CountEnbPort=on  CountDirPort=off  CountDataType=Unsigned  CountWordLen=2  CountFracLen=0  CountSampTime=1/(fs*2)
  Product{,1,3..16} (16 alike) : Product  SaturateOnIntegerOverflow=on
  Product{17..32} (16 alike) : Product
  Product2 : Product  RndMeth=Round  SaturateOnIntegerOverflow=on
  Subsystem : Subsystem
  Subsystem1 : Subsystem
  Subsystem2 : Subsystem
  Subsystem3 : Subsystem
  Subsystem4 : Subsystem
  Subsystem5 : Subsystem
  Subtract{1..16,19..27,29..35} (32 alike) : Sum  Inputs=+-  OutDataTypeStr=fixdt(1,w+1,f)  SaturateOnIntegerOverflow=on
  Subtract18 : Sum  Inputs=+-  OutDataTypeStr=fixdt(1,(w+1)*2+2,f*2)  SaturateOnIntegerOverflow=on
  sign_extend : Subsystem
  symmetric_saturation : MATLAB Function  TreatAsAtomicUnit=on
  LLR Values : Outport
  wires:
  Bit Slice1/1 -> Data Type Conversion/1
  Bit Slice/1 -> Data Type Conversion1/1
  Data Type Conversion1/1 -> Subtract27/1, Subtract29/1, Subtract30/1, Subtract31/1, Subtract32/1, Subtract33/1, Subtract34/1, Subtract35/1, Subtract20/1, Subtract26/1, Subtract25/1, Subtract24/1, Subtract23/1, Subtract22/1, Subtract21/1, Subtract19/1
  Data Type Conversion/1 -> Subtract15/1, Subtract16/1, Subtract14/1, Subtract13/1, Subtract12/1, Subtract11/1, Subtract10/1, Subtract9/1, Subtract7/1, Subtract8/1, Subtract6/1, Subtract5/1, Subtract4/1, Subtract1/1, Subtract3/1, Subtract2/1
  sign_extend/1(y) -> LLR Values/1
  Product2/1 -> symmetric_saturation/1(u)
  symmetric_saturation/1(y) -> sign_extend/1(u)
  HDL Counter/1 -> Subsystem3/1(enb), Subsystem/1(enb), Subsystem4/1(enb), Subsystem5/1(enb)
  valid/1 -> HDL Counter/1
  Subsystem/8(Out8) -> Subtract26/2
  Subsystem/7(Out7) -> Subtract25/2
  Subsystem/6(Out6) -> Subtract24/2
  Subsystem/5(Out5) -> Subtract23/2
  Subsystem/4(Out4) -> Subtract22/2
  Subsystem/3(Out3) -> Subtract21/2
  Subsystem/2(Out2) -> Subtract20/2
  Subsystem/1(Out1) -> Subtract19/2
  Subtract6/1 -> Product19/2, Product19/1
  Subtract22/1 -> Product24/2, Product24/1
  Subtract20/1 -> Product26/1, Product26/2
  Subtract7/1 -> Product18/2, Product18/1
  Subtract8/1 -> Product17/1, Product17/2
  Subtract27/1 -> Product16/2, Product16/1
  Subtract29/1 -> Product15/2, Product15/1
  Subtract30/1 -> Product14/2, Product14/1
  Subtract31/1 -> Product13/2, Product13/1
  Subtract32/1 -> Product12/2, Product12/1
  Subtract33/1 -> Product11/2, Product11/1
  Subtract14/1 -> Product3/2, Product3/1
  Subsystem5/5(Out5) -> Subtract31/2
  Subtract16/1 -> Product/1, Product/2
  Add5/1 -> Subsystem2/5(a2)
  Subsystem3/8(Out8) -> Subtract8/2
  Add4/1 -> Subsystem2/4(b1)
  Product11/1 -> Add10/2
  Product29/1 -> Add4/1
  Subsystem4/8(Out8) -> Subtract16/2
  Subsystem4/2(Out2) -> Subtract10/2
  Subsystem5/8(Out8) -> Subtract27/2
  Subsystem5/7(Out7) -> Subtract29/2
  Subtract11/1 -> Product6/1, Product6/2
  Subtract34/1 -> Product10/1, Product10/2
  Product32/1 -> Add1/1
  Subsystem5/1(Out1) -> Subtract35/2
  Subtract12/1 -> Product5/1, Product5/2
  Subsystem3/7(Out7) -> Subtract7/2
  Product16/1 -> Add15/2
  Subsystem4/1(Out1) -> Subtract9/2
  Subsystem5/6(Out6) -> Subtract30/2
  Product24/1 -> Add4/2
  Subtract3/1 -> Product31/2, Product31/1
  Product13/1 -> Add12/2
  Subsystem5/3(Out3) -> Subtract33/2
  Subsystem5/2(Out2) -> Subtract34/2
  Subsystem4/3(Out3) -> Subtract11/2
  Product17/1 -> Add8/1
  Subsystem4/4(Out4) -> Subtract12/2
  Product9/1 -> Add16/2
  Add9/1 -> Subsystem1/2(b)
  Subsystem4/7(Out7) -> Subtract15/2
  Subtract26/1 -> Product20/2, Product20/1
  Subsystem3/3(Out3) -> Subtract1/2
  Product28/1 -> Add5/1
  Product12/1 -> Add11/2
  Product8/1 -> Add16/1
  Product7/1 -> Add9/1
  Subsystem4/5(Out5) -> Subtract13/2
  Subsystem3/4(Out4) -> Subtract4/2
  Product21/1 -> Add7/2
  Subtract25/1 -> Product21/2, Product21/1
  Add6/1 -> Subsystem2/6(b2)
  Add11/1 -> Subsystem1/4(b1)
  Add2/1 -> Subsystem2/2(b)
  Product15/1 -> Add14/2
  Product14/1 -> Add13/2
  Add8/1 -> Subsystem2/8(b3)
  Product27/1 -> Add1/2
  Subsystem3/1(Out1) -> Subtract2/2
  Subtract9/1 -> Product8/1, Product8/2
  Subtract15/1 -> Product1/1, Product1/2
  Subtract23/1 -> Product23/1, Product23/2
  Add14/1 -> Subsystem1/7(a3)
  imag/1 -> Bit Slice1/1  "y"
  Add16/1 -> Subsystem1/1(a)
  Subtract2/1 -> Product32/2, Product32/1
  Subtract5/1 -> Product28/2, Product28/1
  Subtract4/1 -> Product29/1, Product29/2
  Product18/1 -> Add7/1
  Add15/1 -> Subsystem1/8(b3)
  Product30/1 -> Add3/1
  Subsystem3/5(Out5) -> Subtract5/2
  Product31/1 -> Add2/1
  Subtract19/1 -> Product27/2, Product27/1
  Product26/1 -> Add2/2
  Add13/1 -> Subsystem1/6(b2)
  Subsystem3/2(Out2) -> Subtract3/2
  Product22/1 -> Add6/2
  Subsystem1/1(min) -> Subtract18/2
  Product5/1 -> Add11/1
  Subtract18/1 -> Product2/1
  Subsystem4/6(Out6) -> Subtract14/2
  Subtract1/1 -> Product30/2, Product30/1
  Subtract24/1 -> Product22/2, Product22/1
  Add10/1 -> Subsystem1/3(a1)
  LLR Scale/1 -> Product2/2
  Product4/1 -> Add12/1
  Subtract21/1 -> Product25/2, Product25/1
  Product23/1 -> Add5/2
  Add7/1 -> Subsystem2/7(a3)
  Product3/1 -> Add13/1
  Product19/1 -> Add6/1
  Product25/1 -> Add3/2
  real/1 -> Bit Slice/1  "X"
  Subtract35/1 -> Product9/1, Product9/2
  Subtract10/1 -> Product7/1, Product7/2
  Subsystem3/6(Out6) -> Subtract6/2
  Subsystem2/1(min) -> Subtract18/1
  Add3/1 -> Subsystem2/3(a1)
  Product20/1 -> Add8/2
  Add1/1 -> Subsystem2/1(a)
  Product/1 -> Add15/1
  Subtract13/1 -> Product4/2, Product4/1
  Product1/1 -> Add14/1
  Add12/1 -> Subsystem1/5(a2)
  Product10/1 -> Add9/2
  Product6/1 -> Add10/1
  Subsystem5/4(Out4) -> Subtract32/2

== system fec_ber_hw_V2/Soft Demodulation/SSR Soft Demodulation Lane 1/Soft Demodulation 1 ==
  note: zeros
  note: ones
  valid : Inport
  real : Inport  Port=2
  imag : Inport  Port=3
  LLR Scale : Inport  Port=4
  Add{1..16} (16 alike) : Sum  OutDataTypeStr=fixdt(1,(w+1)*2+1,f*2)  SaturateOnIntegerOverflow=on
  Bit Slice : hdlsllib/Logic and Bit Operations/Bit Slice  lidx=(n*w)-1  ridx=(n-1)*w
      settings: SourceProductBaseCode=SL
  Bit Slice1 : hdlsllib/Logic and Bit Operations/Bit Slice  lidx=(n*w)-1  ridx=(n-1)*w
      settings: SourceProductBaseCode=SL
  Data Type Conversion : DataTypeConversion  OutDataTypeStr=fixdt(1,w,f)  ConvertRealWorld=Stored Integer (SI)  SaturateOnIntegerOverflow=on
  Data Type Conversion1 : DataTypeConversion  OutDataTypeStr=fixdt(1,w,f)  ConvertRealWorld=Stored Integer (SI)  SaturateOnIntegerOverflow=on
  HDL Counter : hdlsllib/Sources/HDL Counter  CountType=Count limited  CountInit=0  CountStep=1  CountMax=3  CountFromType=Initial value  CountFrom=0  CountResetPort=off  CountLoadPort=off  CountEnbPort=on  CountDirPort=off  CountDataType=Unsigned  CountWordLen=2  CountFracLen=0  CountSampTime=1/(fs*2)
  Product{,1,3..16} (16 alike) : Product  SaturateOnIntegerOverflow=on
  Product{17..32} (16 alike) : Product
  Product2 : Product  RndMeth=Round  SaturateOnIntegerOverflow=on
  Subsystem : Subsystem
  Subsystem1 : Subsystem
  Subsystem2 : Subsystem
  Subsystem3 : Subsystem
  Subsystem4 : Subsystem
  Subsystem5 : Subsystem
  Subtract{1..16,19..27,29..35} (32 alike) : Sum  Inputs=+-  OutDataTypeStr=fixdt(1,w+1,f)  SaturateOnIntegerOverflow=on
  Subtract18 : Sum  Inputs=+-  OutDataTypeStr=fixdt(1,(w+1)*2+2,f*2)  SaturateOnIntegerOverflow=on
  sign_extend : Subsystem
  symmetric_saturation : MATLAB Function  TreatAsAtomicUnit=on
  LLR Values : Outport
  wires:
  Subsystem5/4(Out4) -> Subtract32/2
  Product6/1 -> Add10/1
  Product10/1 -> Add9/2
  Add12/1 -> Subsystem1/5(a2)
  Product1/1 -> Add14/1
  Subtract13/1 -> Product4/1, Product4/2
  Product/1 -> Add15/1
  Add1/1 -> Subsystem2/1(a)
  Product20/1 -> Add8/2
  Add3/1 -> Subsystem2/3(a1)
  Subsystem2/1(min) -> Subtract18/1
  Subsystem3/6(Out6) -> Subtract6/2
  Subtract10/1 -> Product7/2, Product7/1
  Subtract35/1 -> Product9/2, Product9/1
  real/1 -> Bit Slice/1  "X"
  Product25/1 -> Add3/2
  Product19/1 -> Add6/1
  Product3/1 -> Add13/1
  Add7/1 -> Subsystem2/7(a3)
  Product23/1 -> Add5/2
  Subtract21/1 -> Product25/1, Product25/2
  Product4/1 -> Add12/1
  LLR Scale/1 -> Product2/2
  Add10/1 -> Subsystem1/3(a1)
  Subtract24/1 -> Product22/1, Product22/2
  Subtract1/1 -> Product30/1, Product30/2
  Subsystem4/6(Out6) -> Subtract14/2
  Subtract18/1 -> Product2/1
  Product5/1 -> Add11/1
  Subsystem1/1(min) -> Subtract18/2
  Product22/1 -> Add6/2
  Subsystem3/2(Out2) -> Subtract3/2
  Add13/1 -> Subsystem1/6(b2)
  Product26/1 -> Add2/2
  Subtract19/1 -> Product27/1, Product27/2
  Product31/1 -> Add2/1
  Subsystem3/5(Out5) -> Subtract5/2
  Product30/1 -> Add3/1
  Add15/1 -> Subsystem1/8(b3)
  Product18/1 -> Add7/1
  Subtract4/1 -> Product29/2, Product29/1
  Subtract5/1 -> Product28/1, Product28/2
  Subtract2/1 -> Product32/1, Product32/2
  Add16/1 -> Subsystem1/1(a)
  imag/1 -> Bit Slice1/1  "y"
  Add14/1 -> Subsystem1/7(a3)
  Subtract23/1 -> Product23/2, Product23/1
  Subtract15/1 -> Product1/2, Product1/1
  Subtract9/1 -> Product8/2, Product8/1
  Subsystem3/1(Out1) -> Subtract2/2
  Product27/1 -> Add1/2
  Add8/1 -> Subsystem2/8(b3)
  Product14/1 -> Add13/2
  Product15/1 -> Add14/2
  Add2/1 -> Subsystem2/2(b)
  Add11/1 -> Subsystem1/4(b1)
  Add6/1 -> Subsystem2/6(b2)
  Subtract25/1 -> Product21/1, Product21/2
  Product21/1 -> Add7/2
  Subsystem3/4(Out4) -> Subtract4/2
  Subsystem4/5(Out5) -> Subtract13/2
  Product7/1 -> Add9/1
  Product8/1 -> Add16/1
  Product12/1 -> Add11/2
  Product28/1 -> Add5/1
  Subsystem3/3(Out3) -> Subtract1/2
  Subtract26/1 -> Product20/1, Product20/2
  Subsystem4/7(Out7) -> Subtract15/2
  Add9/1 -> Subsystem1/2(b)
  Product9/1 -> Add16/2
  Subsystem4/4(Out4) -> Subtract12/2
  Product17/1 -> Add8/1
  Subsystem4/3(Out3) -> Subtract11/2
  Subsystem5/2(Out2) -> Subtract34/2
  Subsystem5/3(Out3) -> Subtract33/2
  Product13/1 -> Add12/2
  Subtract3/1 -> Product31/1, Product31/2
  Product24/1 -> Add4/2
  Subsystem5/6(Out6) -> Subtract30/2
  Subsystem4/1(Out1) -> Subtract9/2
  Product16/1 -> Add15/2
  Subsystem3/7(Out7) -> Subtract7/2
  Subtract12/1 -> Product5/2, Product5/1
  Subsystem5/1(Out1) -> Subtract35/2
  Product32/1 -> Add1/1
  Subtract34/1 -> Product10/2, Product10/1
  Subtract11/1 -> Product6/2, Product6/1
  Subsystem5/7(Out7) -> Subtract29/2
  Subsystem5/8(Out8) -> Subtract27/2
  Subsystem4/2(Out2) -> Subtract10/2
  Subsystem4/8(Out8) -> Subtract16/2
  Product29/1 -> Add4/1
  Product11/1 -> Add10/2
  Add4/1 -> Subsystem2/4(b1)
  Subsystem3/8(Out8) -> Subtract8/2
  Add5/1 -> Subsystem2/5(a2)
  Subtract16/1 -> Product/2, Product/1
  Subsystem5/5(Out5) -> Subtract31/2
  Subtract14/1 -> Product3/1, Product3/2
  Subtract33/1 -> Product11/1, Product11/2
  Subtract32/1 -> Product12/1, Product12/2
  Subtract31/1 -> Product13/1, Product13/2
  Subtract30/1 -> Product14/1, Product14/2
  Subtract29/1 -> Product15/1, Product15/2
  Subtract27/1 -> Product16/1, Product16/2
  Subtract8/1 -> Product17/2, Product17/1
  Subtract7/1 -> Product18/1, Product18/2
  Subtract20/1 -> Product26/2, Product26/1
  Subtract22/1 -> Product24/1, Product24/2
  Subtract6/1 -> Product19/1, Product19/2
  Subsystem/1(Out1) -> Subtract19/2
  Subsystem/2(Out2) -> Subtract20/2
  Subsystem/3(Out3) -> Subtract21/2
  Subsystem/4(Out4) -> Subtract22/2
  Subsystem/5(Out5) -> Subtract23/2
  Subsystem/6(Out6) -> Subtract24/2
  Subsystem/7(Out7) -> Subtract25/2
  Subsystem/8(Out8) -> Subtract26/2
  valid/1 -> HDL Counter/1
  HDL Counter/1 -> Subsystem5/1(enb), Subsystem4/1(enb), Subsystem/1(enb), Subsystem3/1(enb)
  symmetric_saturation/1(y) -> sign_extend/1(u)
  Product2/1 -> symmetric_saturation/1(u)
  sign_extend/1(y) -> LLR Values/1
  Data Type Conversion/1 -> Subtract2/1, Subtract3/1, Subtract1/1, Subtract4/1, Subtract5/1, Subtract6/1, Subtract8/1, Subtract7/1, Subtract9/1, Subtract10/1, Subtract11/1, Subtract12/1, Subtract13/1, Subtract14/1, Subtract16/1, Subtract15/1
  Data Type Conversion1/1 -> Subtract19/1, Subtract21/1, Subtract22/1, Subtract23/1, Subtract24/1, Subtract25/1, Subtract26/1, Subtract20/1, Subtract35/1, Subtract34/1, Subtract33/1, Subtract32/1, Subtract31/1, Subtract30/1, Subtract29/1, Subtract27/1
  Bit Slice/1 -> Data Type Conversion1/1
  Bit Slice1/1 -> Data Type Conversion/1
